simulink model "ECE486_drive_OpenL"  (R2018b)
settings: Solver=ode1  StartTime=0.0  StopTime=50  FixedStep=0.01  RelTol=1e-3  EnableMultiTasking=on
libraries: gtbox x6, simulink x3
settings Model: SimulationMode=external  ExtModeTrigDuration=200000  Creator=David  LastModifiedBy=optiplex3060
settings DataIOCC: LimitDataPoints=on  SaveFormat=Array  SignalLoggingSaveFormat=ModelDataLogs
settings OptimizationCC: ExpressionDepthLimit=2147483647
settings DebuggingCC: UnderspecifiedInitializationDetection=Classic  MergeDetectMultiDrivingBlocksExec=none  SolverPrmCheckMsg=warning  FcnCallInpInsideContextMsg=warning  StateNameClashWarn=warning  SFUnexpectedBacktrackingDiag=warning  SFNoUnconditionalDefaultTransitionDiag=warning  SFExecutionAtInitializationDiag=none
settings ModelReferenceCC: PropagateSignalLabelsOutOfModel=off
settings SFSimCC: SimUseLocalCustomCode=off
settings RTWCC: SystemTargetFile=sldrt.tlc  TemplateMakefile=sldrt.tmf  Description=Simulink Desktop Real-Time  RTWUseLocalCustomCode=off  RTWCompilerOptimization=on
settings CodeAppCC: MaxIdLength=95  StateflowObjectComments=on
settings SimulinkDesktopRealTimeCC: TargetPreCompLibLocation=E:\Program Files\MATLAB\R2018b\toolbox\sldrt\lib\win64  TargetLangStandard=C89/C90 (ANSI)  SupportVariableSizeSignals=off  PreserveStateflowLocalDataDimensions=off
settings ConfigComp: CovMetricSettings=dw  CovHtmlReporting=on  CovSaveCumulativeToWorkspaceVar=on  CovSaveSingleToWorkspaceVar=on  CovExternalEMLEnable=off

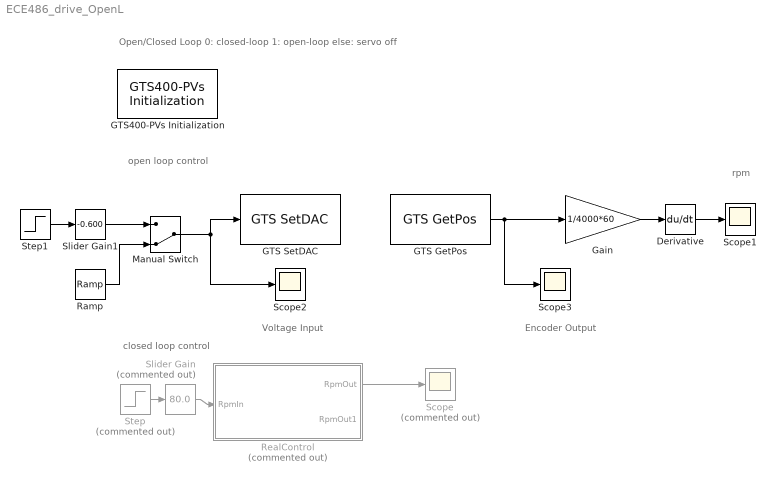
== system ECE486_drive_OpenL ==
  note: Encoder Output
  note: Voltage Input
  note: Open/Closed Loop 0: closed-loop 1: open-loop else: servo off
  note: open loop control
  note: closed loop control
  note: rpm
  Derivative : Derivative
  GTS GetPos : gtbox/GTS-400-PV Function Blocks/GTS GetPos  axis=2
      settings: SourceProductName=Googol Education Products v2.0
  GTS SetDAC : gtbox/GTS-400-PV Function Blocks/GTS SetDAC  Priority=1  port=2
      settings: SourceProductName=Googol Education Products v2.0
  GTS400-PVs Initialization : gtbox/GTS-400-PV Function Blocks/GTS400-PVs Initialization  Priority=0  open=1  mode=0  servo=[0 1 0 0]  aft=[0 0 0 0]  pid1=[1 0 0]  pid2=[1 0 0]  pid3=[1 0 0]  pid4=[1 0 0]  enc1=off  enc2=on  enc3=off  enc4=off  lmt1=off  lmt2=off  lmt3=off  lmt4=off  cdno=2
      settings: SourceProductName=Googol Education Products v2.0
  Gain : Gain  Gain=1/4000*60
  Manual Switch : ManualSwitch  CurrentSetting=0
  Ramp : simulink/Sources/Ramp  slope=.1  start=0  InitialOutput=0
  RealControl : Subsystem  Commented=on
      mask Display:
      | disp('Motor');
      | port_label('input', 1, 'RpmIn');
      | port_label('Output', 1, 'RpmOut');
  Scope : Scope  Commented=on
  Scope1 : Scope
  Scope2 : Scope
  Scope3 : Scope
  Slider Gain : simulink/Math Operations/Slider Gain  Commented=on  gain=80.0  low=-1000  high=2000
  Slider Gain1 : simulink/Math Operations/Slider Gain  gain=-0.600  low=-10  high=10
  Step : Step  Commented=on  SampleTime=0
  Step1 : Step  SampleTime=0
  wires:
  RealControl/1(RpmOut) -> Scope/1
  Step/1 -> Slider Gain/1
  Slider Gain/1 -> RealControl/1(RpmIn)
  Step1/1 -> Slider Gain1/1
  Derivative/1 -> Scope1/1
  Gain/1 -> Derivative/1
  GTS GetPos/1 -> Scope3/1, Gain/1
  Slider Gain1/1 -> Manual Switch/1
  Manual Switch/1 -> GTS SetDAC/1, Scope2/1
  Ramp/1 -> Manual Switch/2

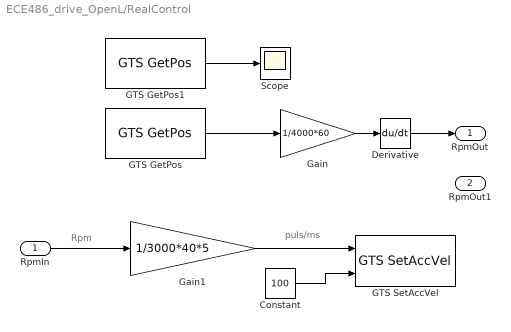
== system ECE486_drive_OpenL/RealControl ==
  note: Rpm
  note: puls/ms
  RpmIn : Inport
  Constant : Constant  Value=100
  Derivative : Derivative
  GTS GetPos : gtbox/GTS-400-PV Function Blocks/GTS GetPos  axis=2
      settings: SourceProductName=Googol Education Products v2.0
  GTS GetPos1 : gtbox/GTS-400-PV Function Blocks/GTS GetPos  axis=1
      settings: SourceProductName=Googol Education Products v2.0
  GTS SetAccVel : gtbox/GTS-400-PV Function Blocks/GTS SetAccVel  Axis=2  vel=0.1  pos=250000000000
      settings: SourceProductName=Googol Education Products v2.0
  Gain : Gain  Gain=1/4000*60
  Gain1 : Gain  Gain=1/3000*40*5
  Scope : Scope
  RpmOut : Outport
  RpmOut1 : Outport  Port=2
  wires:
  RpmIn/1 -> Gain1/1
  Gain/1 -> Derivative/1
  GTS GetPos/1 -> Gain/1
  Gain1/1 -> GTS SetAccVel/1
  Constant/1 -> GTS SetAccVel/2
  GTS GetPos1/1 -> Scope/1
  Derivative/1 -> RpmOut/1
